simulink model "model"  (Simulink 7.6)
settings: Solver=ode45  StartTime=0.0  StopTime=10.0  RelTol=1e-3
values from neighbouring files (symbols this model uses):
  a1 = 0.000001    (= 1e-06)    [main.m]
  a2 = 0.000001    (= 1e-06)    [main.m]
  freq1 = freq2    (= 2)    [main.m]
  freq2 = 2    [main.m]
  g = 9.81    [main.m]    (also in main_BB.m; main_single_BFGS.m; rownania.m = 9; sim_1e-7_error.mat)
  I = 2/5*M*R^2    (= 3.6e-08)    [main.m]    (also in main_BB.m; main_single_BFGS.m; sim_1e-7_error.mat; sim_20steps.mat)
  M = 0.040    (= 0.04)    [main.m]    (also in main_BB.m; main_single_BFGS.m; sim_1e-7_error.mat; sim_20steps.mat)
  phi1 = 3*pi/2    (= 4.71238898038)    [main.m]
  phi2 = 0*pi/2    (= 0)    [main.m]
  R = 0    [BFGS.m]    (also in main.m = 0.0015)
  x0 = [0, 0, 0.00000005, 0,0,-0.0000005]    [main.m]    (also in main_BB.m = [0.1 0 0 0 0.1 0 0 0 0]; main_single_BFGS.m = [0.1 0 0 0 0.1 0 0 0 0]; rownania.m = [0;0;0;0;0;0]; sim_1e-7_error.mat = [0.1 0 0 0 0.1 0 0 0 0])
settings Model: Creator=Dzientak  LastModifiedBy=Dzientak

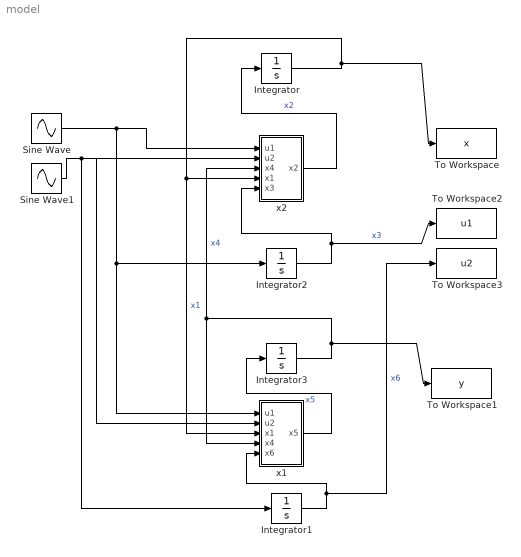
== system model ==
  Integrator : Integrator  InitialCondition=x0(1)
  Integrator1 : Integrator  InitialCondition=x0(6)
  Integrator2 : Integrator  InitialCondition=x0(3)
  Integrator3 : Integrator  InitialCondition=x0(4)
  Sine Wave : Sin  Amplitude=a1  Frequency=freq1  Phase=phi1  SampleTime=0
  Sine Wave1 : Sin  Amplitude=a2  Frequency=freq2  Phase=phi2  SampleTime=0
  To Workspace : ToWorkspace  VariableName=x  SampleTime=-1  SaveFormat=Array
  To Workspace1 : ToWorkspace  VariableName=y  SampleTime=-1  SaveFormat=Array
  To Workspace2 : ToWorkspace  VariableName=u1  SampleTime=-1  SaveFormat=Array
  To Workspace3 : ToWorkspace  VariableName=u2  SampleTime=-1  SaveFormat=Array
  x1 : Subsystem
  x2 : Subsystem
  wires:
  x2/1(x2) -> Integrator/1  "x2"
  Integrator/1 -> x2/4(x1), x1/3(x1), To Workspace/1  "x1"
  Integrator2/1 -> x2/5(x3), To Workspace2/1  "x3"
  Integrator3/1 -> x2/3(x4), x1/4(x4), To Workspace1/1  "x4"
  Sine Wave/1 -> x2/1(u1), Integrator2/1, x1/1(u1)
  Sine Wave1/1 -> x1/2(u2), x2/2(u2), Integrator1/1
  x1/1(x5) -> Integrator3/1  "x5"
  Integrator1/1 -> x1/5(x6), To Workspace3/1  "x6"

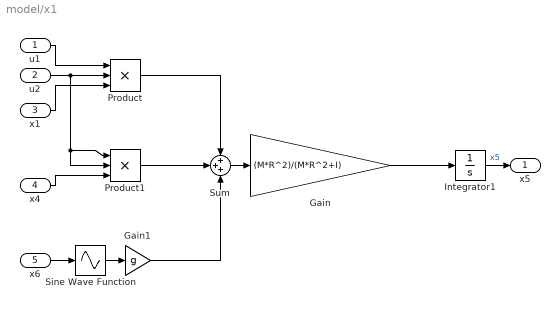
== system model/x1 ==
  u1 : Inport
  u2 : Inport  Port=2
  x1 : Inport  Port=3
  x4 : Inport  Port=4
  x6 : Inport  Port=5
  Gain : Gain  Gain=(M*R^2)/(M*R^2+I)
  Gain1 : Gain  Gain=g
  Integrator1 : Integrator  InitialCondition=x0(5)
  Product : Product  Inputs=3  RndMeth=Zero
  Product1 : Product  Inputs=3  RndMeth=Zero
  Sine Wave Function : Sin  TimeSource=Use external signal  SampleTime=0
  Sum : Sum  Inputs=+++
  x5 : Outport
  wires:
  x6/1 -> Sine Wave Function/1
  x4/1 -> Product1/3
  Integrator1/1 -> x5/1  "x5"
  x1/1 -> Product/3
  u2/1 -> Product/2, Product1/2, Product1/1
  u1/1 -> Product/1
  Gain1/1 -> Sum/3
  Product1/1 -> Sum/2
  Sine Wave Function/1 -> Gain1/1
  Product/1 -> Sum/1
  Gain/1 -> Integrator1/1
  Sum/1 -> Gain/1

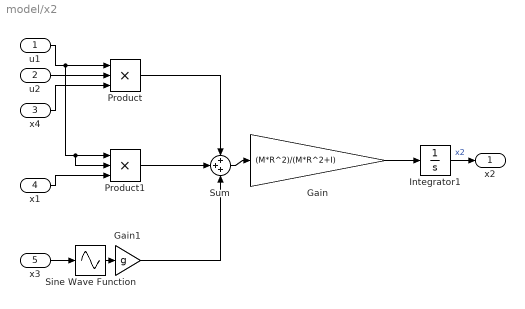
== system model/x2 ==
  u1 : Inport
  u2 : Inport  Port=2
  x4 : Inport  Port=3
  x1 : Inport  Port=4
  x3 : Inport  Port=5
  Gain : Gain  Gain=(M*R^2)/(M*R^2+I)
  Gain1 : Gain  Gain=g
  Integrator1 : Integrator  InitialCondition=x0(2)
  Product : Product  Inputs=3  RndMeth=Zero
  Product1 : Product  Inputs=3  RndMeth=Zero
  Sine Wave Function : Sin  TimeSource=Use external signal  SampleTime=0
  Sum : Sum  Inputs=+++
  x2 : Outport
  wires:
  Sum/1 -> Gain/1
  Gain/1 -> Integrator1/1
  Product/1 -> Sum/1
  Sine Wave Function/1 -> Gain1/1
  Product1/1 -> Sum/2
  Gain1/1 -> Sum/3
  u1/1 -> Product/1, Product1/1, Product1/2
  u2/1 -> Product/2
  x4/1 -> Product/3
  Integrator1/1 -> x2/1  "x2"
  x1/1 -> Product1/3
  x3/1 -> Sine Wave Function/1
